simulink model "newBLDCmodel"  (R2019a)
settings: Solver=VariableStepAuto  StartTime=0.0  StopTime=3  MaxStep=.001  RelTol=1e-3
libraries: simulink x1
settings Model: Creator=tdarrah  LastModifiedBy=darrahts
settings SolverCC: InitialStep=.001  ShapePreserveControl=EnableAll
settings DataIOCC: ReturnWorkspaceOutputs=off
settings DebuggingCC: ArithmeticOperatorsInVariantConditions=warning
settings SFSimCC: SimUseLocalCustomCode=off
settings RTWCC: RTWUseLocalCustomCode=off
settings CodeAppCC: StateflowObjectComments=on

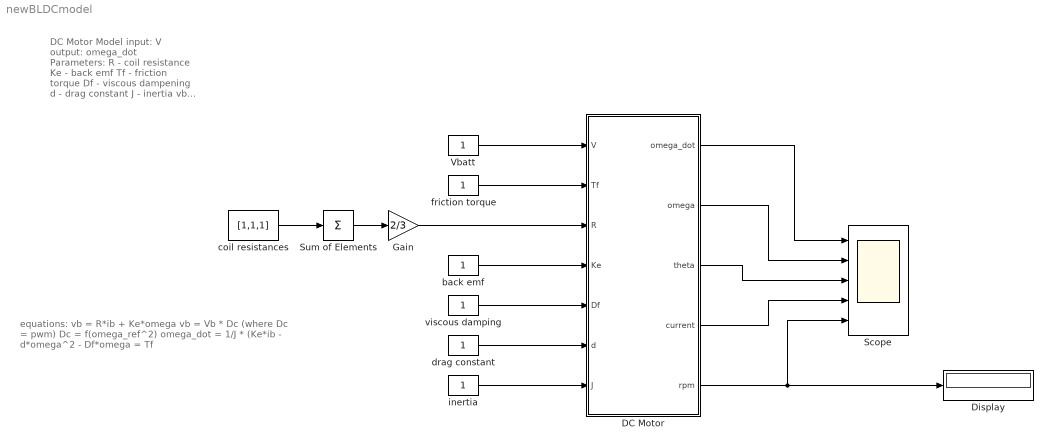
== system newBLDCmodel ==
  note: equations:
      |
      | vb = R*ib + Ke*omega
      | vb = Vb * Dc  (where Dc = pwm)
      | Dc = f(omega_ref^2)
      |
      | omega_dot = 1/J * (Ke*ib - d*omega^2 - Df*omega = Tf
  note: DC Motor Model
      |
      | input:
      | V
      |
      | output:
      | omega_dot
      |
      | Parameters:
      | R   - coil resistance
      | Ke - back emf
      | Tf  - friction torque
      | Df  - viscous dampening
      | d   - drag constant
      | J   - inertia
      | vb - average battery voltage
      | ib  - average battery current
  DC Motor : Subsystem
  Display : Display
  Gain : Gain  Gain=2/3
  Scope : Scope  NumInputPorts=5
  Sum of Elements : Sum  Inputs=+
  Vbatt : Constant
  back emf : Constant
  coil resistances : Constant  Value=[1,1,1]
  drag constant : Constant
  friction torque : Constant
  inertia : Constant
  viscous damping : Constant
  wires:
  DC Motor/2(omega) -> Scope/2
  DC Motor/3(theta) -> Scope/3
  DC Motor/5(rpm) -> Scope/5, Display/1
  DC Motor/4(current) -> Scope/4
  DC Motor/1(omega_dot) -> Scope/1
  Sum of Elements/1 -> Gain/1
  coil resistances/1 -> Sum of Elements/1
  Gain/1 -> DC Motor/3(R)
  Vbatt/1 -> DC Motor/1(V)
  friction torque/1 -> DC Motor/2(Tf)
  back emf/1 -> DC Motor/4(Ke)
  viscous damping/1 -> DC Motor/5(Df)
  drag constant/1 -> DC Motor/6(d)
  inertia/1 -> DC Motor/7(J)

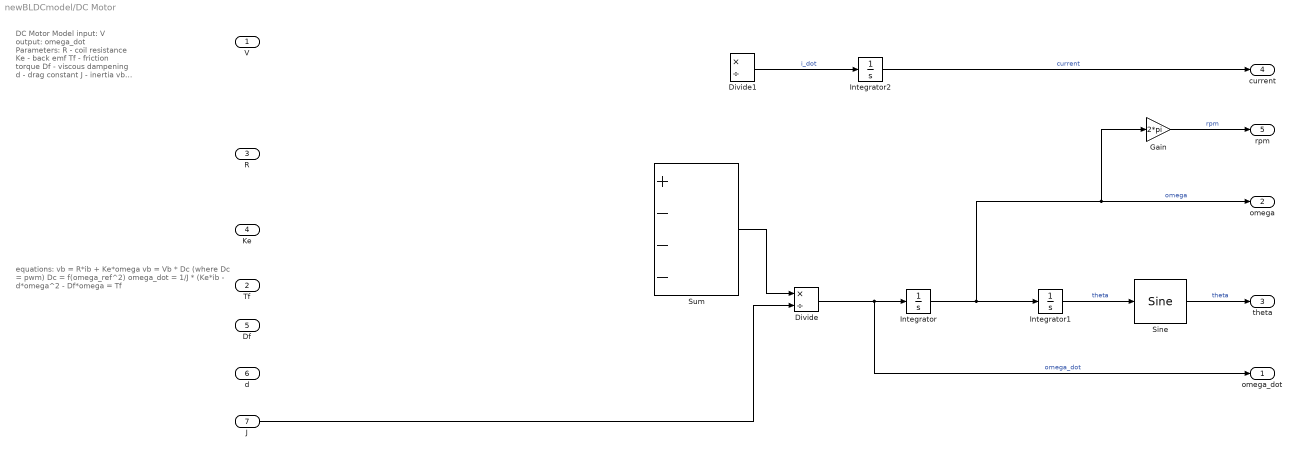
== system newBLDCmodel/DC Motor ==
  note: DC Motor Model
      |
      | input:
      | V
      |
      | output:
      | omega_dot
      |
      | Parameters:
      | R   - coil resistance
      | Ke - back emf
      | Tf  - friction torque
      | Df  - viscous dampening
      | d   - drag constant
      | J   - inertia
      |
      |
      | vb - average battery voltage
      | ib  - average battery current
  note: equations:
      |
      | vb = R*ib + Ke*omega
      | vb = Vb * Dc  (where Dc = pwm)
      | Dc = f(omega_ref^2)
      |
      | omega_dot = 1/J * (Ke*ib - d*omega^2 - Df*omega = Tf
  V : Inport
  Tf : Inport  Port=2
  R : Inport  Port=3
  Ke : Inport  Port=4
  Df : Inport  Port=5
  d : Inport  Port=6
  J : Inport  Port=7
  Divide : Product  Inputs=*/
  Divide1 : Product  Inputs=*/
  Gain : Gain  Gain=2*pi
  Integrator : Integrator
  Integrator1 : Integrator
  Integrator2 : Integrator
  Sine : simulink/Lookup Tables/Sine  Formula=sin(2*pi*u)  NumDataPoints=180  OutputWordLength=16  InternalRulePriority=Speed
      settings: SourceProductName=Simulink
  Sum : Sum  Inputs=+---
  omega_dot : Outport
  omega : Outport  Port=2
  theta : Outport  Port=3
  current : Outport  Port=4
  rpm : Outport  Port=5
  wires:
  Divide/1 -> omega_dot/1, Integrator/1  "omega_dot"
  Integrator/1 -> Gain/1, omega/1, Integrator1/1  "omega"
  Integrator2/1 -> current/1  "current"
  Integrator1/1 -> Sine/1  "theta"
  Divide1/1 -> Integrator2/1  "i_dot"
  Sine/1 -> theta/1  "theta"
  Gain/1 -> rpm/1  "rpm"
  Sum/1 -> Divide/1
  J/1 -> Divide/2
